simulink model "Arduino_Control_Level"  (R2024b)
settings: Solver=FixedStepAuto  StartTime=0.0  StopTime=1000  FixedStep=0.5  RelTol=1e-3  EnableMultiTasking=on
values from neighbouring files (symbols this model uses):
  C = 6.8    [Arduino_Control_Script.m]    (also in PI_Level_Control_Script.m)
  k = 0.032    [Arduino_Control_Script.m]    (also in PI_Level_Control_Script.m)
  k1 = 0.624    [Arduino_Control_Script.m]    (also in PI_Level_Control_Script.m)
  k2 = -0.015    [Arduino_Control_Script.m]    (also in PI_Level_Control_Script.m)
  k3 = -0.0006    [Arduino_Control_Script.m]    (also in PI_Level_Control_Script.m)
  keta = 8*10^-5    (= 8e-05)    [Arduino_Control_Script.m]    (also in PI_Level_Control_Script.m)
libraries: instrumentseriallib x3, svdutilitieslib x2, slpidlib x1
settings Model: Creator=Octavian  LastModifiedBy=Octavian

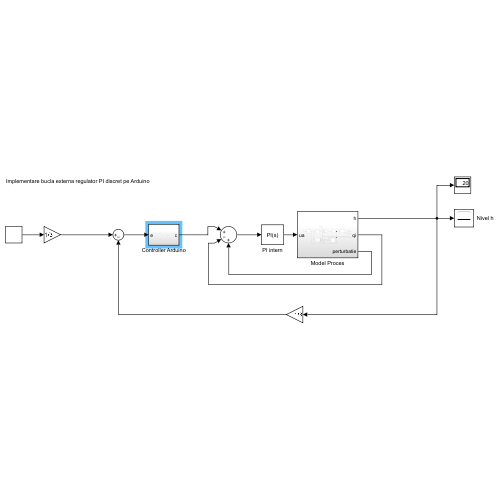
[thumbnail: Simulink's stored preview of the top-level diagram]
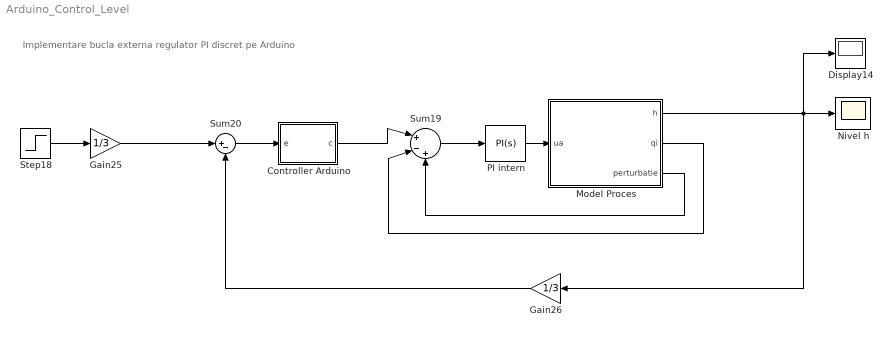
== system Arduino_Control_Level ==
  note: Implementare bucla externa regulator PI discret pe Arduino
  Controller Arduino : Subsystem
  Display14 : Display
  Gain25 : Gain  Gain=1/3
  Gain26 : Gain  Gain=1/3
  Model Proces : Subsystem
  Nivel h : Scope
  PI intern : slpidlib/PID Controller  Controller=PI  Form=Parallel  TimeDomain=Continuous-time  UseExternalTs=off  SampleTime=-1  IntegratorMethod=Forward Euler  FilterMethod=Forward Euler  ControllerParametersSource=internal  P=0.256  I=0.256*1/0.79  UseKiTs=off  D=0  UseExternalDerivativeSource=off  N=100  UseFilter=on  TunerSelectOption=Transfer Function Based (PID Tuner App)  InitialConditionSource=internal  InitialConditionForIntegrator=5.2  InitialConditionForFilter=0  DifferentiatorICPrevScaledInput=0  ExternalReset=none  TrackingMode=off  Kt=1  LimitOutput=off  SatLimitsSource=internal  UpperSaturationLimit=inf  LowerSaturationLimit=-inf  LinearizeAsGain=on  AntiWindupMode=none  Kb=1  LimitIntegrator=off  UpperIntegratorSaturationLimit=inf  LowerIntegratorSaturationLimit=-inf  POutMin=[]  POutMax=[]  IOutMin=[]  IOutMax=[]  DOutMin=[]  DOutMax=[]  NOutMin=[]  NOutMax=[]  SumOutMin=[]  SumOutMax=[]  SaturationOutMin=[]  SaturationOutMax=[]  PParamMin=[]  PParamMax=[]  IParamMin=[]  IParamMax=[]  DParamMin=[]  DParamMax=[]  NParamMin=[]  NParamMax=[]  KbParamMin=[]  KbParamMax=[]  KtParamMin=[]  KtParamMax=[]  KbOutMin=[]  KbOutMax=[]  KtOutMin=[]  KtOutMax=[]  IntegratorOutMin=[]  IntegratorOutMax=[]  FilterOutMin=[]  FilterOutMax=[]  SumI1OutMin=[]  SumI1OutMax=[]  SumI2OutMin=[]  SumI2OutMax=[]  SumI3OutMin=[]  SumI3OutMax=[]  SumI4OutMin=[]  SumI4OutMax=[]  SumDOutMin=[]  SumDOutMax=[]  DifferentiatorOutMin=[]  DifferentiatorOutMax=[]  FilterDiffOutCoefMin=[]  FilterDiffOutCoefMax=[]  ReciprocalOutMin=[]  ReciprocalOutMax=[]  SumDenOutMin=[]  SumDenOutMax=[]  SumNumOutMin=[]  SumNumOutMax=[]  DivideOutMin=[]  DivideOutMax=[]  UdiffTsProdOutMin=[]  UdiffTsProdOutMax=[]  NTsProdOutMin=[]  NTsProdOutMax=[]  UintegralTsProdOutMin=[]  UintegralTsProdOutMax=[]  UngainTsProdOutMin=[]  UngainTsProdOutMax=[]  ClampingZeroOutDataTypeStr=Inherit: Inherit via back propagation  ClampingZeroOutMin=[]  ClampingZeroOutMax=[]  FilterDenConstantOutDataTypeStr=Inherit: Inherit via back propagation  FilterDenConstantOutMin=[]  FilterDenConstantOutMax=[]  PCopyOutDataTypeStr=Inherit: Inherit via back propagation  PCopyOutMin=[]  PCopyOutMax=[]  NCopyOutDataTypeStr=Inherit: Inherit via back propagation  NCopyOutMin=[]  NCopyOutMax=[]  IntegratorContinuousStateAttributes=''  IntegratorStateMustResolveToSignalObject=off  IntegratorRTWStateStorageClass=Auto  FilterContinuousStateAttributes=''  FilterStateMustResolveToSignalObject=off  FilterRTWStateStorageClass=Auto  ParallelPVariant=InternalParameters  IdealPVariant=Disabled  IVariant=InternalParameters  DVariant=Disabled  IntegratorVariant=Continuous  SatVariant=Disabled  AWVariant=Passthrough  PCopyVariant=Disabled  TRVariant=Disabled  FdbkBlocksVariant=Forward  IdealPFdbkVariant=Disabled  SatFdbkVariant=Disabled  DerivativeFilterVariant=Disabled  NVariant=Disabled  NCopyVariant=Disabled_SignalSpec  FilterICVariant=Disabled  IntegratorICVariant=InternalICs  ExternalResetVariant=Disabled  TRSumVariant=Passthrough  SumFdbkVariant=Disabled  SumVariant=Sum_PI  TsampFilterVariant=InternalTs  TsampNgainVariant=Passthrough  TsampIntegralVariant=Disabled_SignalSpec  ExternalSaturationOutDataTypeStr=Inherit: Same as second input  DerivativeSourceVariant=Disabled  PreIntVariant=InternalPreInt
  Step18 : Step  Time=0  After=20  SampleTime=0
  Sum19 : Sum  Inputs=|+-+
  Sum20 : Sum  Inputs=|+-
  wires:
  Model Proces/2(qi) -> Sum19/2
  Gain26/1 -> Sum20/2
  Model Proces/1(h) -> Gain26/1, Nivel h/1, Display14/1
  Step18/1 -> Gain25/1
  Gain25/1 -> Sum20/1
  Model Proces/3(perturbatie) -> Sum19/3
  PI intern/1 -> Model Proces/1(ua)
  Sum19/1 -> PI intern/1
  Sum20/1 -> Controller Arduino/1(e)
  Controller Arduino/1(c) -> Sum19/1

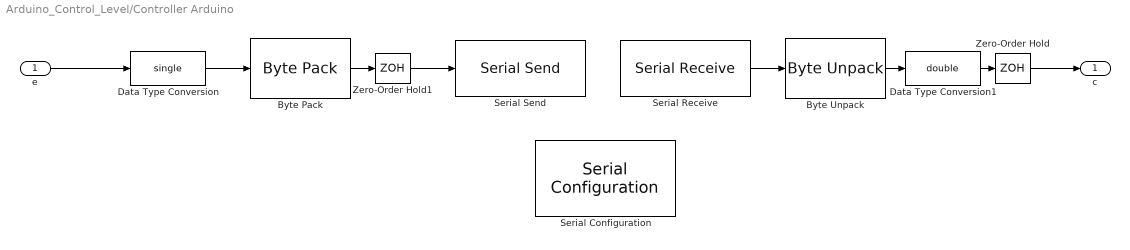
== system Arduino_Control_Level/Controller Arduino ==
  e : Inport
  Byte Pack : svdutilitieslib/Byte Pack  maskPackedDataType=uint8  datatypes={'single'}  byteAlign=1  blockPlatform=arduinoert
  Byte Unpack : svdutilitieslib/Byte Unpack  dimensions={[1]}  datatypes={'single'}  byteAlign=1  blockPlatform=arduinoert
  Data Type Conversion : DataTypeConversion  OutDataTypeStr=single  SaturateOnIntegerOverflow=off  RndMeth=Floor
  Data Type Conversion1 : DataTypeConversion  OutDataTypeStr=double  SaturateOnIntegerOverflow=off  RndMeth=Floor
  Serial Configuration : instrumentseriallib/Serial Configuration  Priority=-200000  PortSel=COM5  Port=COM5  ComPort=COM5  BaudRate=19200  DataBits=8  Parity=none  StopBits=1  ByteOrder=little-endian  FlowControl=none  Timeout=10  SimulateUsing=Interpreted execution  BlockInModel=on  aMode=1
  Serial Receive : instrumentseriallib/Serial Receive  Priority=1  PortSel=COM5  Port=COM5  ComPort=COM5  DataType=uint8  SaveDataType=uint8  ToggleHeader=off  Header=[]  ToggleDataSize=on  DataSize=[4 1]  ToggleTerminator=off  Terminator=<none>  CustomTerminator=[]  InputFormat=Column major  EnableBlockingMode=on  ActionDataUnavailable=Output last received value  ActionWhenDataUnavailable=Output last received value  CustomValue=0  SampleTime=0.5  SimulateUsing=Interpreted execution  BlockInModel=on  aMode=1
  Serial Send : instrumentseriallib/Serial Send  Priority=1  PortSel=COM5  Port=COM5  ComPort=COM5  Header=[]  Terminator=<none>  CustomTerminator=[]  EnableBlockingMode=on  SimulateUsing=Interpreted execution  BlockInModel=on  aMode=1
  Zero-Order Hold : ZeroOrderHold  SampleTime=0.5
  Zero-Order Hold1 : ZeroOrderHold  SampleTime=0.5
  c : Outport
  wires:
  Zero-Order Hold1/1 -> Serial Send/1
  e/1 -> Data Type Conversion/1
  Byte Pack/1 -> Zero-Order Hold1/1
  Zero-Order Hold/1 -> c/1
  Serial Receive/1 -> Byte Unpack/1
  Byte Unpack/1 -> Data Type Conversion1/1
  Data Type Conversion1/1 -> Zero-Order Hold/1
  Data Type Conversion/1 -> Byte Pack/1

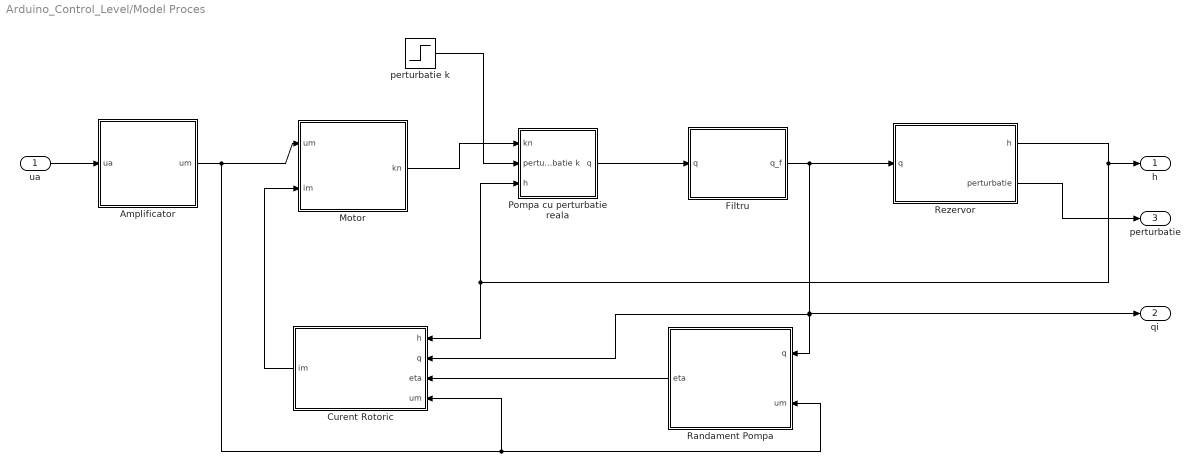
== system Arduino_Control_Level/Model Proces ==
  ua : Inport
  Amplificator : Subsystem
  Curent Rotoric : Subsystem
  Filtru : Subsystem
  Motor : Subsystem
  Pompa cu perturbatie reala : Subsystem
  Randament Pompa : Subsystem
  Rezervor : Subsystem
  perturbatie k : Step  Time=450  After=0.1*k  SampleTime=0
  h : Outport
  qi : Outport  Port=2
  perturbatie : Outport  Port=3
  wires:
  Randament Pompa/1(eta) -> Curent Rotoric/3(eta)
  Rezervor/1(h) -> Pompa cu perturbatie reala/3(h), Curent Rotoric/1(h), h/1
  Curent Rotoric/1(im) -> Motor/2(im)
  Amplificator/1(um) -> Motor/1(um), Randament Pompa/2(um), Curent Rotoric/4(um)
  ua/1 -> Amplificator/1(ua)
  Pompa cu perturbatie reala/1(q) -> Filtru/1(q)
  Motor/1(kn) -> Pompa cu perturbatie reala/1(kn)
  Filtru/1(q_f) -> Randament Pompa/1(q), Curent Rotoric/2(q), qi/1, Rezervor/1(q)
  perturbatie k/1 -> Pompa cu perturbatie reala/2(perturbatie k)
  Rezervor/2(perturbatie) -> perturbatie/1

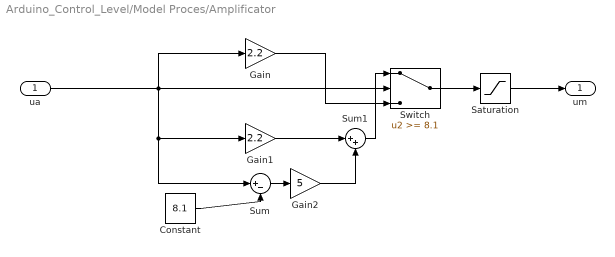
== system Arduino_Control_Level/Model Proces/Amplificator ==
  ua : Inport
  Constant : Constant  Value=8.1
  Gain : Gain  Gain=2.2
  Gain1 : Gain  Gain=2.2
  Gain2 : Gain  Gain=5
  Saturation : Saturate  UpperLimit=22  LowerLimit=0
  Sum : Sum  Inputs=|+-
  Sum1 : Sum  Inputs=|++
  Switch : Switch  Threshold=8.1  SaturateOnIntegerOverflow=off  InputSameDT=off
  um : Outport
  wires:
  ua/1 -> Gain/1, Sum/1, Gain1/1, Switch/2
  Gain1/1 -> Sum1/1
  Gain/1 -> Switch/3
  Sum1/1 -> Switch/1
  Gain2/1 -> Sum1/2
  Constant/1 -> Sum/2
  Switch/1 -> Saturation/1
  Sum/1 -> Gain2/1
  Saturation/1 -> um/1

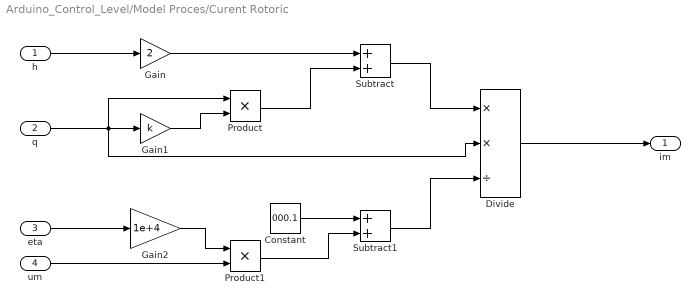
== system Arduino_Control_Level/Model Proces/Curent Rotoric ==
  h : Inport
  q : Inport  Port=2
  eta : Inport  Port=3
  um : Inport  Port=4
  Constant : Constant  Value=000.1
  Divide : Product  Inputs=**/
  Gain : Gain  Gain=2
  Gain1 : Gain  Gain=k
  Gain2 : Gain  Gain=1e+4
  Product : Product
  Product1 : Product
  Subtract : Sum
  Subtract1 : Sum
  im : Outport
  wires:
  Divide/1 -> im/1
  Subtract1/1 -> Divide/3
  Constant/1 -> Subtract1/1
  Gain2/1 -> Product1/1
  q/1 -> Divide/2, Product/1, Gain1/1
  Subtract/1 -> Divide/1
  Product/1 -> Subtract/2
  Gain/1 -> Subtract/1
  Gain1/1 -> Product/2
  Product1/1 -> Subtract1/2
  um/1 -> Product1/2
  h/1 -> Gain/1
  eta/1 -> Gain2/1

== system Arduino_Control_Level/Model Proces/Filtru ==
  q : Inport
  Integrator : Integrator  InitialCondition=27.3  LimitOutput=on  LowerSaturationLimit=0
  Sum : Sum  Inputs=|+-
  q_f : Outport
  wires:
  Sum/1 -> Integrator/1
  Integrator/1 -> q_f/1, Sum/2
  q/1 -> Sum/1

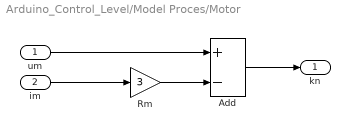
== system Arduino_Control_Level/Model Proces/Motor ==
  um : Inport
  im : Inport  Port=2
  Add : Sum  Inputs=+-
  Rm : Gain  Gain=3
  kn : Outport
  wires:
  Rm/1 -> Add/2
  um/1 -> Add/1
  im/1 -> Rm/1
  Add/1 -> kn/1

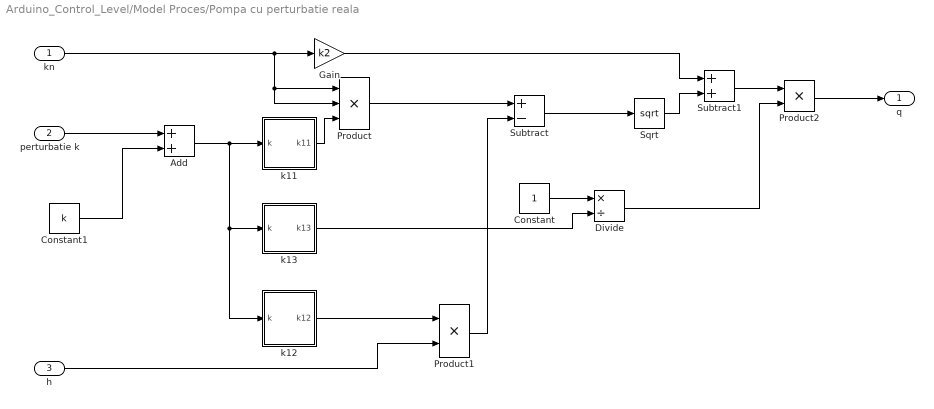
== system Arduino_Control_Level/Model Proces/Pompa cu perturbatie reala ==
  kn : Inport
  perturbatie k : Inport  Port=2
  h : Inport  Port=3
  Add : Sum
  Constant : Constant
  Constant1 : Constant  Value=k
  Divide : Product  Inputs=*/
  Gain : Gain  Gain=k2
  Product : Product  Inputs=3
  Product1 : Product
  Product2 : Product
  Sqrt : Sqrt
  Subtract : Sum  Inputs=+-
  Subtract1 : Sum
  k11 : Subsystem
  k12 : Subsystem
  k13 : Subsystem
  q : Outport
  wires:
  h/1 -> Product1/2
  k12/1(k12) -> Product1/1
  Constant1/1 -> Add/2
  Add/1 -> k12/1(k), k13/1(k), k11/1(k)
  Gain/1 -> Subtract1/1
  Product/1 -> Subtract/1
  Divide/1 -> Product2/2
  kn/1 -> Product/2, Product/1, Gain/1
  Subtract/1 -> Sqrt/1
  k13/1(k13) -> Divide/2
  Subtract1/1 -> Product2/1
  k11/1(k11) -> Product/3
  Constant/1 -> Divide/1
  Product1/1 -> Subtract/2
  Sqrt/1 -> Subtract1/2
  perturbatie k/1 -> Add/1
  Product2/1 -> q/1

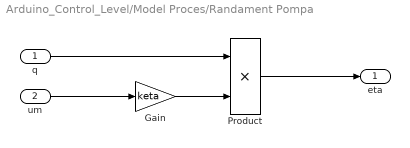
== system Arduino_Control_Level/Model Proces/Randament Pompa ==
  q : Inport
  um : Inport  Port=2
  Gain : Gain  Gain=keta
  Product : Product
  eta : Outport
  wires:
  Gain/1 -> Product/2
  Product/1 -> eta/1
  q/1 -> Product/1
  um/1 -> Gain/1

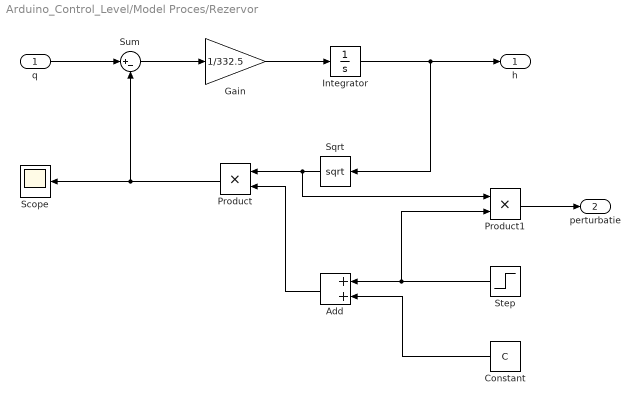
== system Arduino_Control_Level/Model Proces/Rezervor ==
  q : Inport
  Add : Sum
  Constant : Constant  Value=C
  Gain : Gain  Gain=1/332.5
  Integrator : Integrator  InitialCondition=16.02
  Product : Product
  Product1 : Product
  Scope : Scope
  Sqrt : Sqrt
  Step : Step  Time=550  After=2  SampleTime=0
  Sum : Sum  Inputs=|+-
  h : Outport
  perturbatie : Outport  Port=2
  wires:
  Gain/1 -> Integrator/1
  Integrator/1 -> Sqrt/1, h/1
  Sum/1 -> Gain/1
  q/1 -> Sum/1
  Sqrt/1 -> Product1/1, Product/1
  Product/1 -> Scope/1, Sum/2
  Step/1 -> Product1/2, Add/1
  Constant/1 -> Add/2
  Add/1 -> Product/2
  Product1/1 -> perturbatie/1

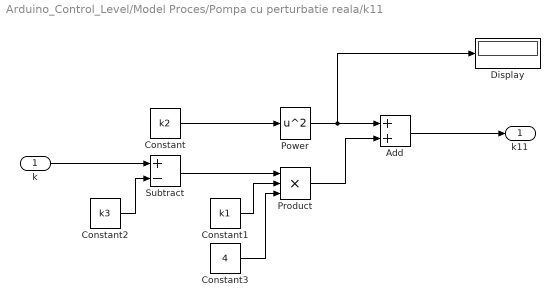
== system Arduino_Control_Level/Model Proces/Pompa cu perturbatie reala/k11 ==
  k : Inport
  Add : Sum
  Constant : Constant  Value=k2
  Constant1 : Constant  Value=k1
  Constant2 : Constant  Value=k3
  Constant3 : Constant  Value=4
  Display : Display
  Power : Math  Operator=square
  Product : Product  Inputs=3
  Subtract : Sum  Inputs=+-
  k11 : Outport
  wires:
  Constant/1 -> Power/1
  Power/1 -> Display/1, Add/1
  k/1 -> Subtract/1
  Constant2/1 -> Subtract/2
  Subtract/1 -> Product/1
  Constant1/1 -> Product/2
  Constant3/1 -> Product/3
  Product/1 -> Add/2
  Add/1 -> k11/1

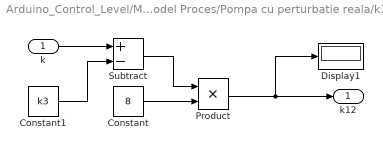
== system Arduino_Control_Level/Model Proces/Pompa cu perturbatie reala/k12 ==
  k : Inport
  Constant : Constant  Value=8
  Constant1 : Constant  Value=k3
  Display1 : Display
  Product : Product
  Subtract : Sum  Inputs=+-
  k12 : Outport
  wires:
  k/1 -> Subtract/1
  Subtract/1 -> Product/1
  Constant1/1 -> Subtract/2
  Constant/1 -> Product/2
  Product/1 -> k12/1, Display1/1

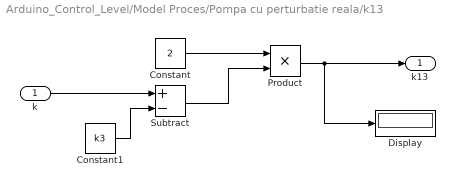
== system Arduino_Control_Level/Model Proces/Pompa cu perturbatie reala/k13 ==
  k : Inport
  Constant : Constant  Value=2
  Constant1 : Constant  Value=k3
  Display : Display
  Product : Product
  Subtract : Sum  Inputs=+-
  k13 : Outport
  wires:
  k/1 -> Subtract/1
  Constant/1 -> Product/1
  Constant1/1 -> Subtract/2
  Subtract/1 -> Product/2
  Product/1 -> k13/1, Display/1
